simulink model "UIO_IMECE"  (R2019b)
settings: Solver=VariableStepAuto  StartTime=0.0  StopTime=25  FixedStep=0.002  RelTol=1e-3
values from neighbouring files (symbols this model uses):
  A = Am+B*Lx*C    [IMECE_UIO_2021_06_08.m]
  Am = [-7 2 4; -2 -1 2;-2 2 -1]    [IMECE_UIO_2021_06_08.m]
  B = [0;0.7;2]    [IMECE_UIO_2021_06_08.m]
  C = [0.5 0 1]    [IMECE_UIO_2021_06_08.m]
  Fu = [0 0 0 0 0;0 0 1 0 0;0 -4 0 0 0;0 0 0 0 1;0 0 0 -16 0]    [IMECE_UIO_2021_06_08.m]
  g1 = 2    [IMECE_UIO_2021_06_08.m]
  g2 = 0    [IMECE_UIO_2021_06_08.m]
  g3 = 0    [IMECE_UIO_2021_06_08.m]
  g4 = 4    [IMECE_UIO_2021_06_08.m]
  g_missing = 0    [IMECE_UIO_2021_06_08.m]
  g_step = 3    [IMECE_UIO_2021_06_08.m]
  gamma_e = 1*ones(size(C,1),1)    [IMECE_UIO_2021_06_08.m]
  Ku = Klqr(length(Am)+1:end,:)    [IMECE_UIO_2021_06_08.m]
  Kx = Klqr(1:length(Am),:)    [IMECE_UIO_2021_06_08.m]
  Theta = ones(size(B,2),size(Fu,1))    [IMECE_UIO_2021_06_08.m]
libraries: dspmtrx3 x1
settings Model: Creator=Tris  LastModifiedBy=Tris

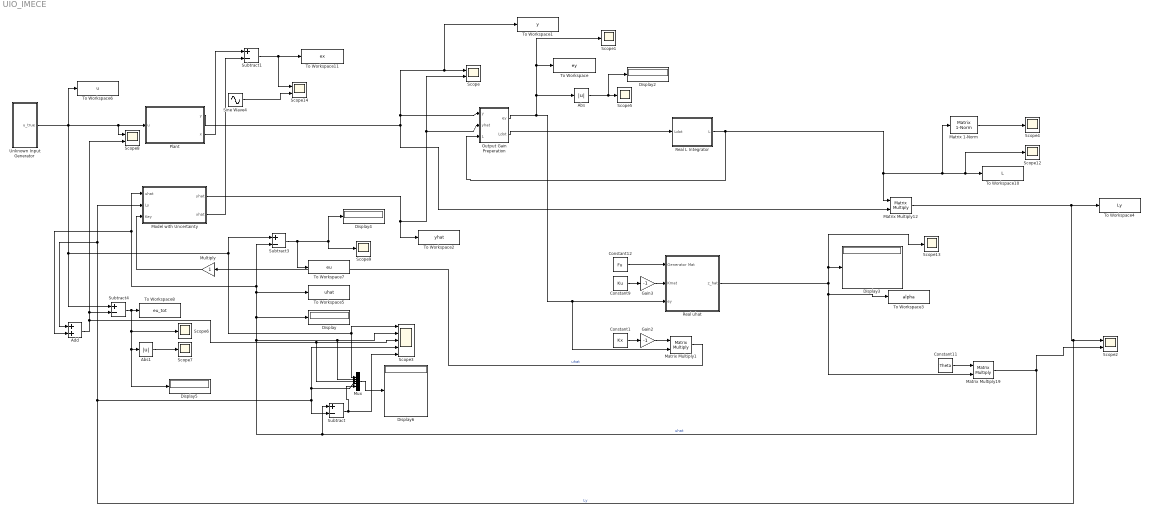
== system UIO_IMECE ==
  Abs : Abs  ZeroCross=off
  Abs1 : Abs
  Add : Sum
  Constant1 : Constant  Value=Kx  VectorParams1D=off
  Constant11 : Constant  Value=Theta  VectorParams1D=off
  Constant12 : Constant  Value=Fu
  Constant9 : Constant  Value=Ku  VectorParams1D=off
  Display{,2..6} (6 alike) : Display
  Gain2 : Gain  Gain=-1
  Gain3 : Gain  Gain=-1
  Matrix 1-Norm : dspmtrx3/Matrix  1-Norm  roundingMode=Floor  overflowMode=off  outputDataTypeStr=Inherit: Same as accumulator  outputMin=[]  outputMax=[]  outputLastDataTypeStr=Inherit: Same as accumulator
      settings: SourceProductName=DSP System Toolbox  SourceProductBaseCode=DS
  Matrix Multiply1 : Product  Multiplication=Matrix(*)
  Matrix Multiply12 : Product  Multiplication=Matrix(*)
  Matrix Multiply19 : Product  Multiplication=Matrix(*)
  Model with Uncertainty : Subsystem
  Multiply : Gain
  Mux : Mux  Inputs=5
  Output Gain Preperation : Subsystem
  Plant : Subsystem
  Real L Integrator : Subsystem
  "Real uhat " : Subsystem
  Scope{,2,8,14} (4 alike) : Scope  NumInputPorts=2
  Scope{1,4..7,9,12..13} (8 alike) : Scope
  Scope3 : Scope  NumInputPorts=5
  Sine Wave4 : Sin  Amplitude=0  Frequency=8  Phase=pi/2  SampleTime=0  VectorParams1D=off
  Subtract{,1,3..4} (4 alike) : Sum  Inputs=+-
  To Workspace : ToWorkspace  VariableName=ey  SaveFormat=Timeseries  SampleTime=-1
  To Workspace1 : ToWorkspace  VariableName=y  SaveFormat=Timeseries  SampleTime=-1
  To Workspace10 : ToWorkspace  VariableName=L  SaveFormat=Timeseries  SampleTime=-1
  To Workspace11 : ToWorkspace  VariableName=ex  SaveFormat=Timeseries  SampleTime=-1
  To Workspace2 : ToWorkspace  VariableName=yhat  SaveFormat=Timeseries  SampleTime=-1
  To Workspace3 : ToWorkspace  VariableName=alpha  SaveFormat=Timeseries  SampleTime=-1
  To Workspace4 : ToWorkspace  VariableName=Ly  SaveFormat=Timeseries  SampleTime=-1
  To Workspace5 : ToWorkspace  VariableName=uhat  SaveFormat=Timeseries  SampleTime=-1
  To Workspace6 : ToWorkspace  VariableName=u  SaveFormat=Timeseries  SampleTime=-1
  To Workspace7 : ToWorkspace  VariableName=eu  SaveFormat=Timeseries  SampleTime=-1
  To Workspace8 : ToWorkspace  VariableName=eu_tot  SaveFormat=Timeseries  SampleTime=-1
  Unknown Input Generator : Subsystem
  wires:
  Constant11/1 -> Matrix Multiply19/1
  Matrix Multiply19/1 -> Subtract/1, Model with Uncertainty/1(uhat), Add/2, Subtract3/2, To Workspace5/1, Display/1, Mux/2, Scope3/2, Scope2/2  "uhat"
  Matrix Multiply12/1 -> To Workspace4/1, Scope3/4, Mux/4, Subtract/2, Model with Uncertainty/2(Ly), Add/1, Scope2/1  "Ly"
  Constant9/1 -> Gain3/1
  Constant12/1 -> "Real uhat "/1(Generator Mat)
  "Real uhat "/1(z_hat) -> To Workspace3/1, Matrix Multiply19/2, Scope13/1, Display3/1
  Plant/1(y) -> To Workspace1/1, Scope/1, Output Gain Preperation/1(y), Matrix Multiply12/2
  Abs/1 -> Display2/1, Scope5/1
  Model with Uncertainty/1(yhat) -> To Workspace2/1, Scope/2, Output Gain Preperation/2(yhat)
  Subtract3/1 -> Display4/1, Scope9/1, To Workspace7/1
  Output Gain Preperation/2(Ldot) -> Real L Integrator/1(Ldot)
  Abs1/1 -> Scope7/1
  Unknown Input Generator/1(u_true) -> Mux/1, Scope3/1, Subtract3/1, Subtract4/1, To Workspace6/1, Scope8/1, Plant/1(u)
  Subtract4/1 -> Display5/1, Abs1/1, Scope6/1, To Workspace8/1
  Matrix 1-Norm/1 -> Scope4/1
  Model with Uncertainty/2(xhat) -> Subtract1/2
  Plant/2(x) -> Subtract1/1
  Subtract1/1 -> Scope14/1, To Workspace11/1
  Sine Wave4/1 -> Scope14/2
  Matrix Multiply1/1 -> Multiply/1  "uhat"
  Constant1/1 -> Gain2/1
  Output Gain Preperation/1(ey) -> To Workspace/1, Scope1/1, Abs/1, Matrix Multiply1/2, "Real uhat "/3(ey)
  Gain2/1 -> Matrix Multiply1/1
  Gain3/1 -> "Real uhat "/2(Kmat)
  Add/1 -> Scope8/2, Subtract4/2, Mux/3, Scope3/3
  Multiply/1 -> Model with Uncertainty/3(Key)
  Mux/1 -> Display6/1
  Subtract/1 -> Mux/5, Scope3/5
  Real L Integrator/1(L) -> Matrix 1-Norm/1, Scope12/1, To Workspace10/1, Matrix Multiply12/1, Output Gain Preperation/3(L)

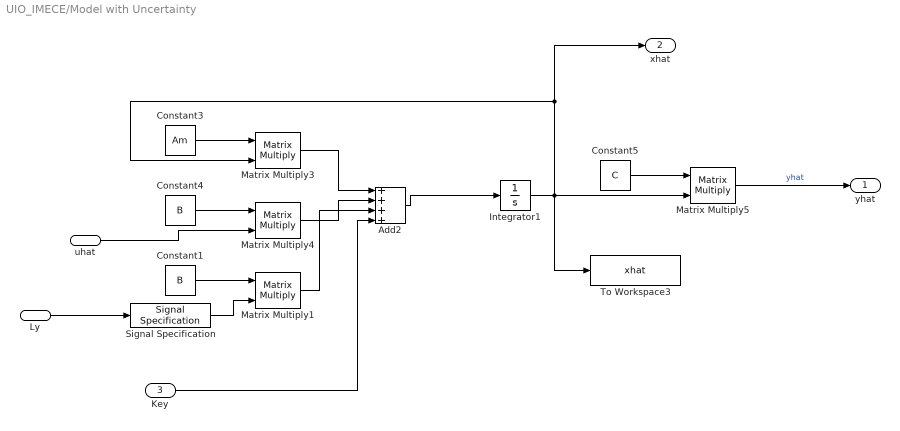
== system UIO_IMECE/Model with Uncertainty ==
  uhat : Inport
  Ly : Inport  Port=2
  Key : Inport  Port=3
  Add2 : Sum  Inputs=++++
  Constant1 : Constant  Value=B  VectorParams1D=off
  Constant3 : Constant  Value=Am
  Constant4 : Constant  Value=B  VectorParams1D=off
  Constant5 : Constant  Value=C  VectorParams1D=off
  Integrator1 : Integrator
  Matrix Multiply{1,3..5} (4 alike) : Product  Multiplication=Matrix(*)
  Signal Specification : SignalSpecification  Dimensions=[1,1]
  To Workspace3 : ToWorkspace  VariableName=xhat  SaveFormat=Timeseries  SampleTime=-1
  yhat : Outport
  xhat : Outport  Port=2
  wires:
  Constant3/1 -> Matrix Multiply3/1
  Integrator1/1 -> To Workspace3/1, Matrix Multiply5/2, xhat/1, Matrix Multiply3/2
  Constant5/1 -> Matrix Multiply5/1
  Add2/1 -> Integrator1/1
  Matrix Multiply4/1 -> Add2/2
  Constant4/1 -> Matrix Multiply4/1
  Matrix Multiply3/1 -> Add2/1
  Matrix Multiply5/1 -> yhat/1  "yhat"
  Key/1 -> Add2/4
  uhat/1 -> Matrix Multiply4/2
  Constant1/1 -> Matrix Multiply1/1
  Ly/1 -> Signal Specification/1
  Matrix Multiply1/1 -> Add2/3
  Signal Specification/1 -> Matrix Multiply1/2

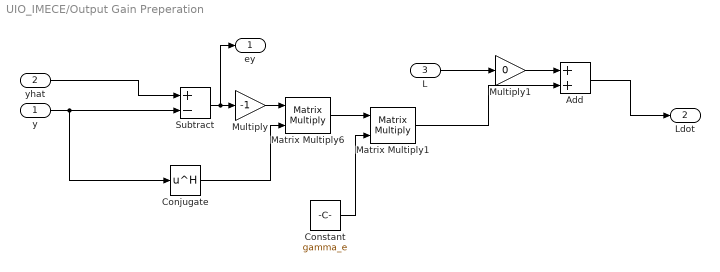
== system UIO_IMECE/Output Gain Preperation ==
  y : Inport
  yhat : Inport  Port=2
  L : Inport  Port=3
  Add : Sum
  Conjugate : Math  Operator=hermitian  RndMeth=Zero  SaturateOnIntegerOverflow=on
  Constant : Constant  Value=gamma_e
  Matrix Multiply1 : Product  Multiplication=Matrix(*)
  Matrix Multiply6 : Product  Multiplication=Matrix(*)
  Multiply : Gain  Gain=-1
  Multiply1 : Gain  Gain=0
  Subtract : Sum  Inputs=+-
  ey : Outport
  Ldot : Outport  Port=2
  wires:
  Matrix Multiply6/1 -> Matrix Multiply1/1
  Multiply/1 -> Matrix Multiply6/1
  Conjugate/1 -> Matrix Multiply6/2
  y/1 -> Subtract/2, Conjugate/1
  yhat/1 -> Subtract/1
  Subtract/1 -> Multiply/1, ey/1
  Constant/1 -> Matrix Multiply1/2
  Add/1 -> Ldot/1
  Matrix Multiply1/1 -> Add/2
  L/1 -> Multiply1/1
  Multiply1/1 -> Add/1

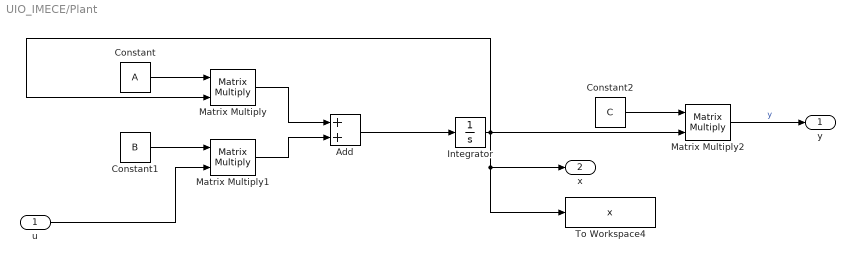
== system UIO_IMECE/Plant ==
  u : Inport
  Add : Sum
  Constant : Constant  Value=A
  Constant1 : Constant  Value=B  VectorParams1D=off
  Constant2 : Constant  Value=C  VectorParams1D=off
  Integrator : Integrator
  Matrix Multiply : Product  Multiplication=Matrix(*)
  Matrix Multiply1 : Product  Multiplication=Matrix(*)
  Matrix Multiply2 : Product  Multiplication=Matrix(*)
  To Workspace4 : ToWorkspace  VariableName=x  SaveFormat=Timeseries  SampleTime=-1
  y : Outport
  x : Outport  Port=2
  wires:
  Constant2/1 -> Matrix Multiply2/1
  Add/1 -> Integrator/1
  Constant1/1 -> Matrix Multiply1/1
  u/1 -> Matrix Multiply1/2
  Matrix Multiply1/1 -> Add/2
  Integrator/1 -> Matrix Multiply/2, x/1, To Workspace4/1, Matrix Multiply2/2
  Constant/1 -> Matrix Multiply/1
  Matrix Multiply/1 -> Add/1
  Matrix Multiply2/1 -> y/1  "y"

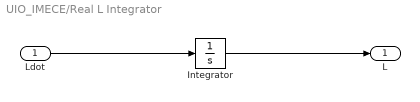
== system UIO_IMECE/Real L Integrator ==
  Ldot : Inport
  Integrator : Integrator  InitialCondition=-8
  L : Outport
  wires:
  Ldot/1 -> Integrator/1
  Integrator/1 -> L/1

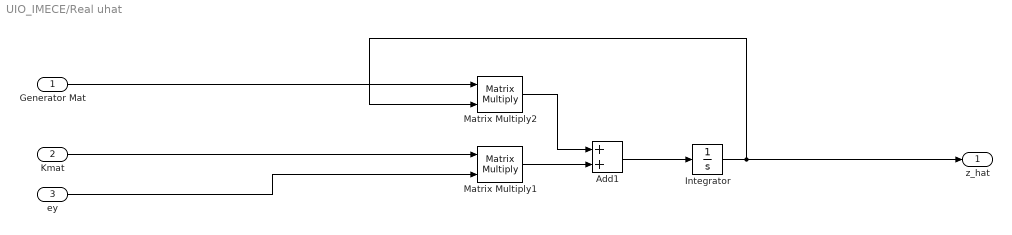
== system UIO_IMECE/Real uhat  ==
  Generator Mat : Inport
  Kmat : Inport  Port=2
  ey : Inport  Port=3
  Add1 : Sum
  Integrator : Integrator  InitialCondition=1
  Matrix Multiply1 : Product  Multiplication=Matrix(*)
  Matrix Multiply2 : Product  Multiplication=Matrix(*)
  z_hat : Outport
  wires:
  ey/1 -> Matrix Multiply1/2
  Generator Mat/1 -> Matrix Multiply2/1
  Kmat/1 -> Matrix Multiply1/1
  Matrix Multiply1/1 -> Add1/2
  Add1/1 -> Integrator/1
  Matrix Multiply2/1 -> Add1/1
  Integrator/1 -> Matrix Multiply2/2, z_hat/1

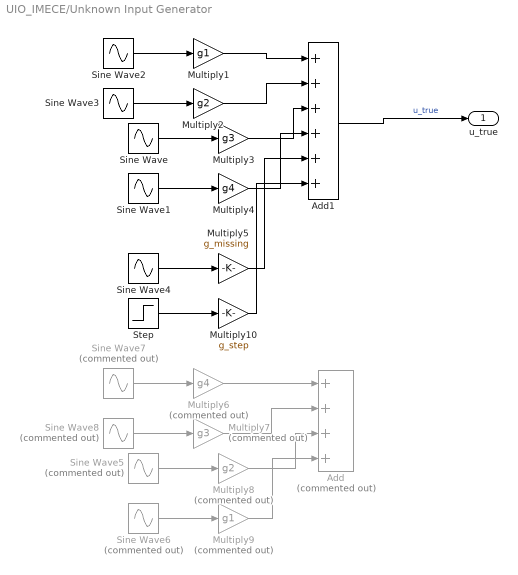
== system UIO_IMECE/Unknown Input Generator ==
  Add : Sum  Commented=on  Inputs=4
  Add1 : Sum  Inputs=++++++
  Multiply1 : Gain  Gain=g1
  Multiply10 : Gain  Gain=g_step
  Multiply2 : Gain  Gain=g2
  Multiply3 : Gain  Gain=g3
  Multiply4 : Gain  Gain=g4
  Multiply5 : Gain  Gain=g_missing
  Multiply6 : Gain  Commented=on  Gain=g4
  Multiply7 : Gain  Commented=on  Gain=g3
  Multiply8 : Gain  Commented=on  Gain=g2
  Multiply9 : Gain  Commented=on  Gain=g1
  Sine Wave : Sin  Frequency=4  SampleTime=0  VectorParams1D=off
  Sine Wave1 : Sin  Frequency=4  Phase=pi/2  SampleTime=0  VectorParams1D=off
  Sine Wave2 : Sin  Frequency=2  SampleTime=0  VectorParams1D=off
  Sine Wave3 : Sin  Frequency=2  Phase=pi/2  SampleTime=0  VectorParams1D=off
  Sine Wave4 : Sin  Frequency=8  Phase=pi/2  SampleTime=0  VectorParams1D=off
  Sine Wave5 : Sin  Commented=on  Frequency=12  SampleTime=0  VectorParams1D=off
  Sine Wave6 : Sin  Commented=on  Frequency=12  Phase=pi/2  SampleTime=0  VectorParams1D=off
  Sine Wave7 : Sin  Commented=on  Frequency=5  SampleTime=0  VectorParams1D=off
  Sine Wave8 : Sin  Commented=on  Frequency=5  Phase=pi/2  SampleTime=0  VectorParams1D=off
  Step : Step  Time=3  SampleTime=0
  u_true : Outport
  wires:
  Multiply4/1 -> Add1/4
  Multiply3/1 -> Add1/3
  Sine Wave/1 -> Multiply3/1
  Sine Wave1/1 -> Multiply4/1
  Multiply2/1 -> Add1/2
  Sine Wave3/1 -> Multiply2/1
  Multiply1/1 -> Add1/1
  Sine Wave2/1 -> Multiply1/1
  Sine Wave4/1 -> Multiply5/1
  Multiply5/1 -> Add1/5
  Multiply6/1 -> Add/1
  Multiply8/1 -> Add/3
  Sine Wave5/1 -> Multiply8/1
  Multiply9/1 -> Add/4
  Multiply7/1 -> Add/2
  Sine Wave7/1 -> Multiply6/1
  Sine Wave8/1 -> Multiply7/1
  Sine Wave6/1 -> Multiply9/1
  Step/1 -> Multiply10/1
  Multiply10/1 -> Add1/6
  Add1/1 -> u_true/1  "u_true"
